simulink model "FTBF_sans_sat"  (R2020a)
settings: Solver=VariableStepAuto  StartTime=0.0  StopTime=0.04  RelTol=1e-3
libraries: cstblocks x3
settings Model: Creator=marche  LastModifiedBy=marche

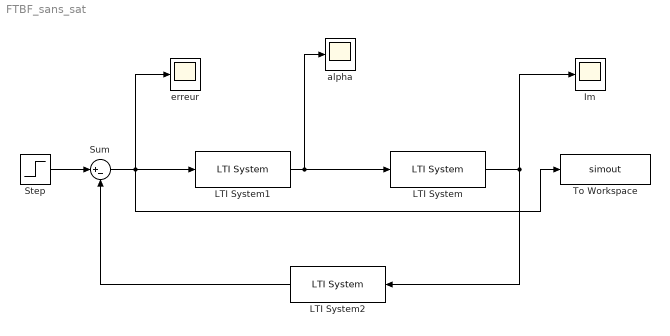
== system FTBF_sans_sat ==
  Im : Scope
  LTI System : cstblocks/LTI System  sys=num  IC=[]
  LTI System1 : cstblocks/LTI System  sys=C  IC=[]
  LTI System2 : cstblocks/LTI System  sys=denum  IC=[]
  Step : Step  Time=0  After=1.65  SampleTime=0
  Sum : Sum  Inputs=|+-
  To Workspace : ToWorkspace  VariableName=simout  SaveFormat=Timeseries  SampleTime=-1
  alpha : Scope
  erreur : Scope
  wires:
  Step/1 -> Sum/1
  Sum/1 -> To Workspace/1, erreur/1, LTI System1/1
  LTI System1/1 -> LTI System/1, alpha/1
  LTI System/1 -> LTI System2/1, Im/1
  LTI System2/1 -> Sum/2
